simulink model "pfd_simulink"  (R2018a)
settings: Solver=ode45  StartTime=0.0  StopTime=0.04  FixedStep=T_ref*0.0001  RelTol=10e-5
values from neighbouring files (symbols this model uses):
  C = 10^-6    (= 1e-06)    [simulation.m]
  I_p = 10^-3    (= 0.001)    [simulation.m]
  initial_filter_state = v_1 - I_p*tau_1/C    (= 10)    [simulation.m]
  initial_ref_phase = 1 + tau_1/T_ref    (= 1)    [simulation.m]
  initial_vco_phase = 0    [simulation.m]
  K_vco = 500    [simulation.m]
  omega_free = 0    [simulation.m]
  R = 1000    [simulation.m]
  T_ref = 10^-3    (= 0.001)    [simulation.m]
settings Model: Creator=mir  LastModifiedBy=mir

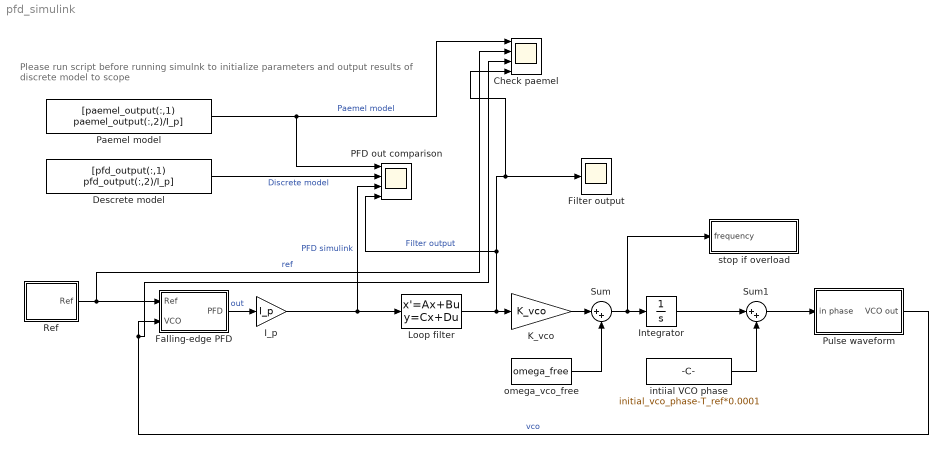
== system pfd_simulink ==
  note: Please run script before running simulnk to initialize parameters
      | and output results of discrete model to scope
  Check paemel : Scope  NumInputPorts=4
  Descrete model : FromWorkspace  VariableName=[pfd_output(:,1) pfd_output(:,2)/I_p]  SampleTime=0
  Falling-edge PFD : Subsystem
  Filter output : Scope
  I_p : Gain  Gain=I_p
  Integrator : Integrator
  K_vco : Gain  Gain=K_vco
  Loop filter : StateSpace  A=0  B=1/C  D=R  InitialCondition=initial_filter_state
  PFD out comparison : Scope  NumInputPorts=4
  Paemel model : FromWorkspace  VariableName=[paemel_output(:,1) paemel_output(:,2)/I_p]  SampleTime=0
  Pulse waveform : Subsystem
  Ref : Subsystem
  Sum : Sum  Inputs=|++
  Sum1 : Sum  Inputs=|++
  intiial VCO phase : Constant  Value=initial_vco_phase-T_ref*0.0001
  omega_vco_free : Constant  Value=omega_free
  stop if overload : Subsystem
  wires:
  I_p/1 -> Loop filter/1, PFD out comparison/3  "PFD simulink"
  Falling-edge PFD/1(PFD) -> I_p/1  "out"
  omega_vco_free/1 -> Sum/2
  Sum/1 -> stop if overload/1(frequency), Integrator/1
  K_vco/1 -> Sum/1
  Loop filter/1 -> PFD out comparison/4, Check paemel/4, Filter output/1, K_vco/1  "Filter output"
  Descrete model/1 -> PFD out comparison/2  "Discrete model"
  intiial VCO phase/1 -> Sum1/2
  Pulse waveform/1(VCO out) -> Check paemel/3, Falling-edge PFD/2(VCO)  "vco"
  Ref/1(Ref) -> Check paemel/2, Falling-edge PFD/1(Ref)  "ref"
  Integrator/1 -> Sum1/1
  Sum1/1 -> Pulse waveform/1(in phase)
  Paemel model/1 -> Check paemel/1, PFD out comparison/1  "Paemel model"

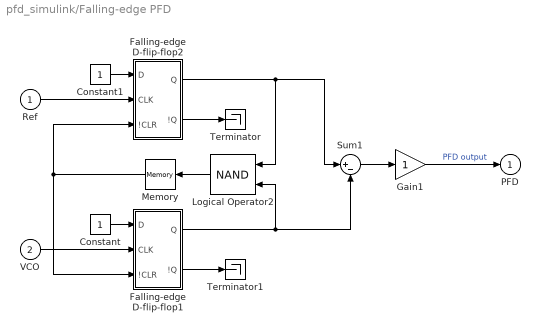
== system pfd_simulink/Falling-edge PFD ==
  Ref : Inport
  VCO : Inport  Port=2
  Constant : Constant  OutDataTypeStr=boolean
  Constant1 : Constant  OutDataTypeStr=boolean
  Falling-edge D-flip-flop1 : Subsystem
  Falling-edge D-flip-flop2 : Subsystem
  Gain1 : Gain  SaturateOnIntegerOverflow=on  OutDataTypeStr=Inherit: Same as input  ParamDataTypeStr=Inherit: Same as input
  Logical Operator2 : Logic  Operator=NAND
  Memory : Memory
  Sum1 : Sum  Inputs=|+-  OutDataTypeStr=double  SaturateOnIntegerOverflow=on  InputSameDT=on
  Terminator : Terminator
  Terminator1 : Terminator
  PFD : Outport  InitialOutput=0
  wires:
  Falling-edge D-flip-flop2/2(!Q) -> Terminator/1
  Logical Operator2/1 -> Memory/1
  Falling-edge D-flip-flop1/1(Q) -> Sum1/2, Logical Operator2/2
  Constant/1 -> Falling-edge D-flip-flop1/1(D)
  Gain1/1 -> PFD/1  "PFD output"
  Ref/1 -> Falling-edge D-flip-flop2/2(CLK)
  Sum1/1 -> Gain1/1
  Falling-edge D-flip-flop1/2(!Q) -> Terminator1/1
  VCO/1 -> Falling-edge D-flip-flop1/2(CLK)
  Memory/1 -> Falling-edge D-flip-flop2/3(!CLR), Falling-edge D-flip-flop1/3(!CLR)
  Constant1/1 -> Falling-edge D-flip-flop2/1(D)
  Falling-edge D-flip-flop2/1(Q) -> Logical Operator2/1, Sum1/1

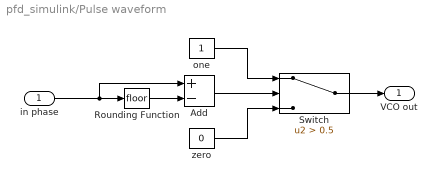
== system pfd_simulink/Pulse waveform ==
  in phase : Inport
  Add : Sum  Inputs=+-
  Rounding Function : Rounding
  Switch : Switch  Criteria=u2 > Threshold  Threshold=0.5
  one : Constant
  zero : Constant  Value=0
  VCO out : Outport
  wires:
  in phase/1 -> Add/1, Rounding Function/1
  Add/1 -> Switch/2
  Rounding Function/1 -> Add/2
  one/1 -> Switch/1
  zero/1 -> Switch/3
  Switch/1 -> VCO out/1

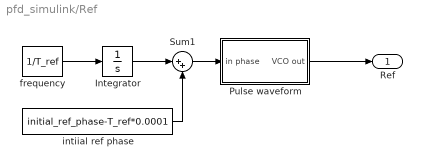
== system pfd_simulink/Ref ==
  Integrator : Integrator
  Pulse waveform : Subsystem
  Sum1 : Sum  Inputs=|++
  frequency : Constant  Value=1/T_ref
  intiial ref phase : Constant  Value=initial_ref_phase-T_ref*0.0001
  Ref : Outport
  wires:
  intiial ref phase/1 -> Sum1/2
  Integrator/1 -> Sum1/1
  Sum1/1 -> Pulse waveform/1(in phase)
  Pulse waveform/1(VCO out) -> Ref/1
  frequency/1 -> Integrator/1

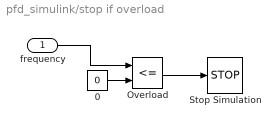
== system pfd_simulink/stop if overload ==
  frequency : Inport
  0 : Constant  Value=0
  Overload : RelationalOperator  Operator=<=  OutDataTypeStr=boolean  RndMeth=Simplest
  Stop Simulation : Stop
  wires:
  frequency/1 -> Overload/1
  Overload/1 -> Stop Simulation/1
  0/1 -> Overload/2

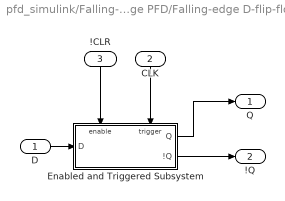
== system pfd_simulink/Falling-edge PFD/Falling-edge D-flip-flop1 ==
  D : Inport
  CLK : Inport  Port=2
  !CLR : Inport  Port=3
  Enabled and Triggered Subsystem : Subsystem  TreatAsAtomicUnit=on
  Q : Outport  InitialOutput=0
  !Q : Outport  Port=2  InitialOutput=1
  wires:
  !CLR/1 -> Enabled and Triggered Subsystem/Enable
  D/1 -> Enabled and Triggered Subsystem/1(D)
  Enabled and Triggered Subsystem/1(Q) -> Q/1
  CLK/1 -> Enabled and Triggered Subsystem/Trigger
  Enabled and Triggered Subsystem/2(!Q) -> !Q/1

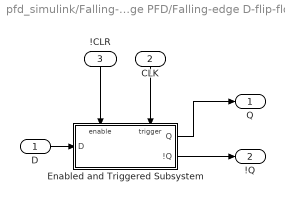
== system pfd_simulink/Falling-edge PFD/Falling-edge D-flip-flop2 ==
  D : Inport
  CLK : Inport  Port=2
  !CLR : Inport  Port=3
  Enabled and Triggered Subsystem : Subsystem  TreatAsAtomicUnit=on
  Q : Outport  InitialOutput=0
  !Q : Outport  Port=2  InitialOutput=1
  wires:
  !CLR/1 -> Enabled and Triggered Subsystem/Enable
  D/1 -> Enabled and Triggered Subsystem/1(D)
  Enabled and Triggered Subsystem/1(Q) -> Q/1
  CLK/1 -> Enabled and Triggered Subsystem/Trigger
  Enabled and Triggered Subsystem/2(!Q) -> !Q/1

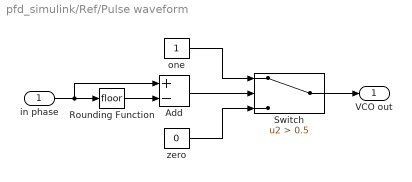
== system pfd_simulink/Ref/Pulse waveform ==
  in phase : Inport
  Add : Sum  Inputs=+-
  Rounding Function : Rounding
  Switch : Switch  Criteria=u2 > Threshold  Threshold=0.5
  one : Constant
  zero : Constant  Value=0
  VCO out : Outport
  wires:
  in phase/1 -> Add/1, Rounding Function/1
  Add/1 -> Switch/2
  Rounding Function/1 -> Add/2
  one/1 -> Switch/1
  zero/1 -> Switch/3
  Switch/1 -> VCO out/1

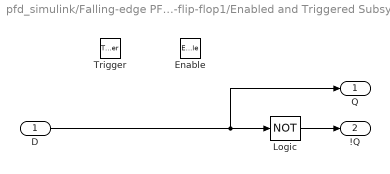
== system pfd_simulink/Falling-edge PFD/Falling-edge D-flip-flop1/Enabled and Triggered Subsystem ==
  D : Inport
  Enable : EnablePort
  Trigger : TriggerPort  TriggerType=falling  VariantControl=Variant
  Logic : Logic  Operator=NOT  Inputs=1
  Q : Outport  OutputWhenDisabled=reset  InitialOutput=0
  !Q : Outport  Port=2  OutputWhenDisabled=reset  InitialOutput=1
  wires:
  D/1 -> Q/1, Logic/1
  Logic/1 -> !Q/1

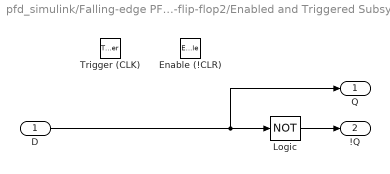
== system pfd_simulink/Falling-edge PFD/Falling-edge D-flip-flop2/Enabled and Triggered Subsystem ==
  D : Inport
  Enable (!CLR) : EnablePort
  Trigger (CLK) : TriggerPort  TriggerType=falling  VariantControl=Variant
  Logic : Logic  Operator=NOT  Inputs=1
  Q : Outport  OutputWhenDisabled=reset  InitialOutput=0
  !Q : Outport  Port=2  OutputWhenDisabled=reset  InitialOutput=1
  wires:
  D/1 -> Q/1, Logic/1
  Logic/1 -> !Q/1
